simulink model "mqsls_sim_3dof_actual"  (R2024b)
settings: configuration reference "prj_default_config" (kept outside this file)
StartFcn:
  | run('control_init.m');
settings Model: Creator=yangyu  LastModifiedBy=yangyu
settings ConfigSetRef: SourceName=prj_default_config  SourceLocation=Base Workspace

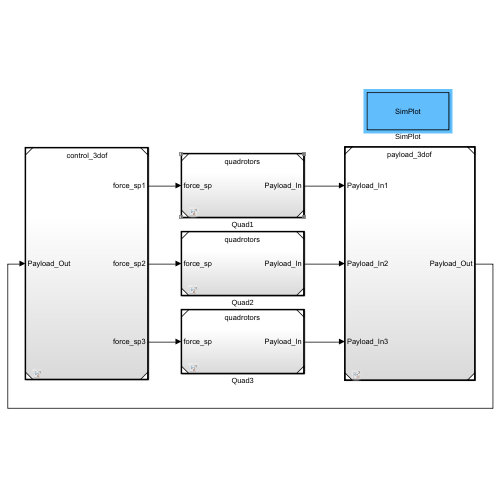
[thumbnail: Simulink's stored preview of the top-level diagram]
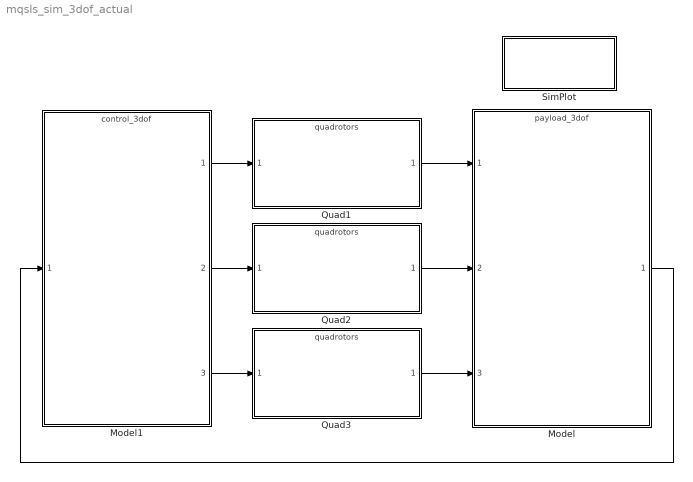
== system mqsls_sim_3dof_actual ==
  Model : ModelReference  ModelNameDialog=payload_3dof  SimulationMode=Normal  ModelReferenceVersion=1.114
  Model1 : ModelReference  ModelNameDialog=control_3dof  SimulationMode=Normal  ModelReferenceVersion=1.484
  Quad1 : ModelReference  ModelNameDialog=quadrotors.slx  SimulationMode=Normal  ModelReferenceVersion=1.84
  Quad2 : ModelReference  ModelNameDialog=quadrotors.slx  SimulationMode=Normal  ModelReferenceVersion=1.84
  Quad3 : ModelReference  ModelNameDialog=quadrotors.slx  SimulationMode=Normal  ModelReferenceVersion=1.84
  SimPlot : Subsystem
      settings: OpenFcn=run('simplot.m');
      mask Display: disp('SimPlot');
  wires:
  Quad3/1 -> Model/3
  Quad2/1 -> Model/2
  Quad1/1 -> Model/1
  Model/1 -> Model1/1
  Model1/1 -> Quad1/1
  Model1/2 -> Quad2/1
  Model1/3 -> Quad3/1

== system mqsls_sim_3dof_actual/SimPlot ==
